simulink model "ejercicio11TAREA_13_02_17"  (R2013a)
settings: Solver=ode45  StartTime=0.0  StopTime=10.0  RelTol=1e-3
libraries: simulink x6
settings Model: Creator=Miguel  LastModifiedBy=Miguel

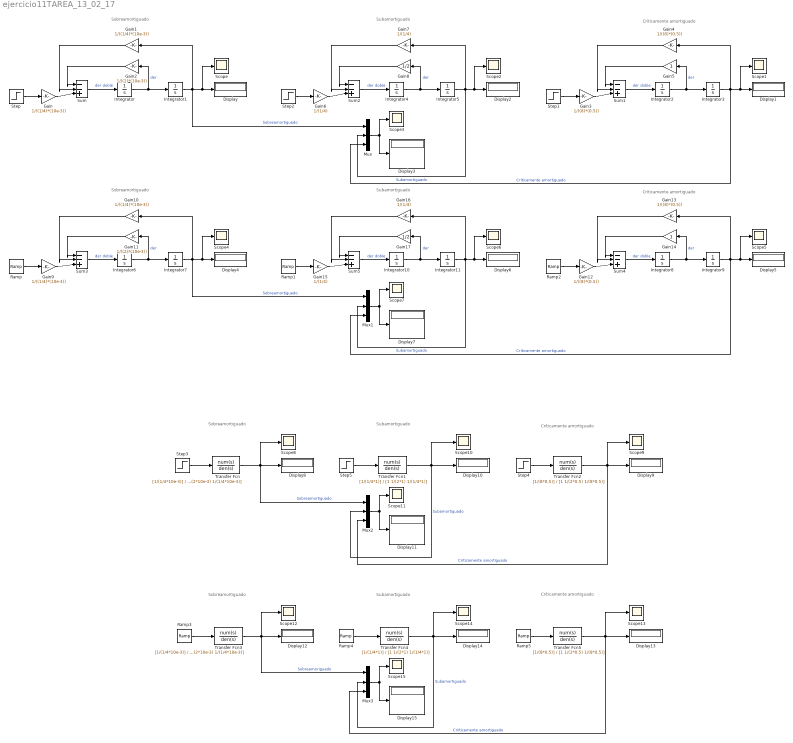
== system ejercicio11TAREA_13_02_17 ==
  note: Críticamente amortiguado
  note: Sobreamortiguado
  note: Subamortiguado
  note: Críticamente amortiguado
  note: Sobreamortiguado
  note: Subamortiguado
  note: Críticamente amortiguado
  note: Sobreamortiguado
  note: Subamortiguado
  note: Críticamente amortiguado
  note: Sobreamortiguado
  note: Subamortiguado
  Display{,1..15} (16 alike) : Display
  Gain{,1,9..10} (4 alike) : Gain  Gain=1/((1/4)*(10e-3))
  Gain11 : Gain  Gain=1/((2)*(10e-3))
  Gain{3..4,12..13} (4 alike) : Gain  Gain=1/((8)*(0.5))
  Gain14 : Gain
  Gain{6..7,15..16} (4 alike) : Gain  Gain=1/(1/4)
  Gain17 : Gain  Gain=1/2
  Gain2 : Gain  Gain=1/((2)*(10e-3))
  Gain5 : Gain
  Gain8 : Gain  Gain=1/2
  Integrator{,1..11} (12 alike) : Integrator
  Mux{,1..3} (4 alike) : Mux  Inputs=3
  Ramp{,1..5} (6 alike) : simulink/Sources/Ramp  slope=1  start=0  X0=0
  Scope{,1..15} (16 alike) : Scope
      Scope10 settings: SaveName=ScopeData8
      Scope11 settings: ShowLegends=on  SaveName=ScopeData9
      Scope12 settings: SaveName=ScopeData10
      Scope13 settings: SaveName=ScopeData11
      Scope14 settings: SaveName=ScopeData12
      Scope15 settings: ShowLegends=on  SaveName=ScopeData13
      Scope2 settings: SaveName=ScopeData2
      Scope3 settings: ShowLegends=on  SaveName=ScopeData3
      Scope4 settings: SaveName=ScopeData4
      Scope5 settings: SaveName=ScopeData5
      Scope6 settings: SaveName=ScopeData6
      Scope7 settings: ShowLegends=on  SaveName=ScopeData7
      Scope8 settings: SaveName=ScopeData14
      Scope9 settings: SaveName=ScopeData15
  Step{,1..5} (6 alike) : Step  SampleTime=0
  Sum{,1..5} (6 alike) : Sum  Inputs=|--+
  Transfer Fcn : TransferFcn  Numerator=[1/(1/4*10e-3)]  Denominator=[1 1/(2*10e-3) 1/(1/4*10e-3)]
  Transfer Fcn1 : TransferFcn  Numerator=[1/(1/4*1)]  Denominator=[1 1/(2*1) 1/(1/4*1)]
  Transfer Fcn2 : TransferFcn  Numerator=[1/(8*0.5)]  Denominator=[1 1/(2*0.5) 1/(8*0.5)]
  Transfer Fcn3 : TransferFcn  Numerator=[1/(1/4*10e-3)]  Denominator=[1 1/(2*10e-3) 1/(1/4*10e-3)]
  Transfer Fcn4 : TransferFcn  Numerator=[1/(1/4*1)]  Denominator=[1 1/(2*1) 1/(1/4*1)]
  Transfer Fcn5 : TransferFcn  Numerator=[1/(8*0.5)]  Denominator=[1 1/(2*0.5) 1/(8*0.5)]
  wires:
  Integrator/1 -> Gain2/1, Integrator1/1  "der"
  Gain/1 -> Sum/3
  Sum/1 -> Integrator/1  "der doble"
  Integrator1/1 -> Mux/1, Display/1, Scope/1, Gain1/1  "Sobreamortiguado"
  Step/1 -> Gain/1
  Gain1/1 -> Sum/2
  Gain2/1 -> Sum/1
  Integrator2/1 -> Gain5/1, Integrator3/1  "der"
  Gain3/1 -> Sum1/3
  Sum1/1 -> Integrator2/1  "der doble"
  Integrator3/1 -> Mux/3, Display1/1, Scope1/1, Gain4/1  "Críticamente amortiguado"
  Step1/1 -> Gain3/1
  Gain4/1 -> Sum1/2
  Gain5/1 -> Sum1/1
  Integrator4/1 -> Gain8/1, Integrator5/1  "der"
  Gain6/1 -> Sum2/3
  Sum2/1 -> Integrator4/1  "der doble"
  Integrator5/1 -> Mux/2, Display2/1, Scope2/1, Gain7/1  "Subamortiguado"
  Step2/1 -> Gain6/1
  Gain7/1 -> Sum2/2
  Gain8/1 -> Sum2/1
  Mux/1 -> Display3/1, Scope3/1
  Integrator6/1 -> Gain11/1, Integrator7/1  "der"
  Gain9/1 -> Sum3/3
  Sum3/1 -> Integrator6/1  "der doble"
  Integrator7/1 -> Mux1/1, Display4/1, Scope4/1, Gain10/1  "Sobreamortiguado"
  Ramp/1 -> Gain9/1
  Gain10/1 -> Sum3/2
  Gain11/1 -> Sum3/1
  Integrator8/1 -> Gain14/1, Integrator9/1  "der"
  Gain12/1 -> Sum4/3
  Sum4/1 -> Integrator8/1  "der doble"
  Integrator9/1 -> Mux1/3, Display5/1, Scope5/1, Gain13/1  "Críticamente amortiguado"
  Ramp2/1 -> Gain12/1
  Gain13/1 -> Sum4/2
  Gain14/1 -> Sum4/1
  Integrator10/1 -> Gain17/1, Integrator11/1  "der"
  Gain15/1 -> Sum5/3
  Sum5/1 -> Integrator10/1  "der doble"
  Integrator11/1 -> Mux1/2, Display6/1, Scope6/1, Gain16/1  "Subamortiguado"
  Ramp1/1 -> Gain15/1
  Gain16/1 -> Sum5/2
  Gain17/1 -> Sum5/1
  Mux1/1 -> Display7/1, Scope7/1
  Step5/1 -> Transfer Fcn1/1
  Mux2/1 -> Display11/1, Scope11/1
  Mux3/1 -> Display15/1, Scope15/1
  Step3/1 -> Transfer Fcn/1
  Transfer Fcn/1 -> Mux2/1, Scope8/1, Display8/1  "Sobreamortiguado"
  Ramp3/1 -> Transfer Fcn3/1
  Transfer Fcn3/1 -> Mux3/1, Scope12/1, Display12/1  "Sobreamoriguado"
  Transfer Fcn1/1 -> Mux2/2, Scope10/1, Display10/1  "Subamortiguado"
  Ramp4/1 -> Transfer Fcn4/1
  Transfer Fcn4/1 -> Mux3/2, Scope14/1, Display14/1  "Subamortiguado"
  Ramp5/1 -> Transfer Fcn5/1
  Step4/1 -> Transfer Fcn2/1
  Transfer Fcn2/1 -> Mux2/3, Scope9/1, Display9/1  "Críticamente amortiguado"
  Transfer Fcn5/1 -> Mux3/3, Scope13/1, Display13/1  "Criíticamente amortiguado"
